simulink model "VentilatorActivity_Start"  (R2024b)
settings: Solver=VariableStepAuto  StartTime=0.0  StopTime=10.0  RelTol=1e-3
model workspace (MAT data in the model file):
  HeatCmd = Simulink.Bus
  HeatCmd.Alignment = -1
  HeatCmd.PreserveElementDimensions = 0
  HeatCmd.Elements_internal = Simulink.BusElement
  HeatCmd.Elements_internal.DimensionsMode = 'Fixed'
  HeatCmd.Elements_internal.SamplingMode = 'Sample based'
  HeatCmd.Elements_internal.SampleTime = -1
  HeatCmd.Elements_internal.Name = 'Element'
  HeatCmd.Elements_internal.DataType_internal = 'double'
  HeatCmd.Elements_internal.Complexity = 'real'
  HeatCmd.Elements_internal.Dimensions = 1
  HeatCmd.DataScope = 'Auto'
  HeaterCmd = Simulink.Bus
  HeaterCmd.Alignment = -1
  HeaterCmd.PreserveElementDimensions = 0
  HeaterCmd.DataScope = 'Auto'
  HumidSens = Simulink.Bus
  HumidSens.Alignment = -1
  HumidSens.PreserveElementDimensions = 0
  HumidSens.DataScope = 'Auto'
  init = Simulink.Bus
  init.Alignment = -1
  init.PreserveElementDimensions = 0
  init.DataScope = 'Auto'
settings Model: Creator=ppatel  LastModifiedBy=ppatel

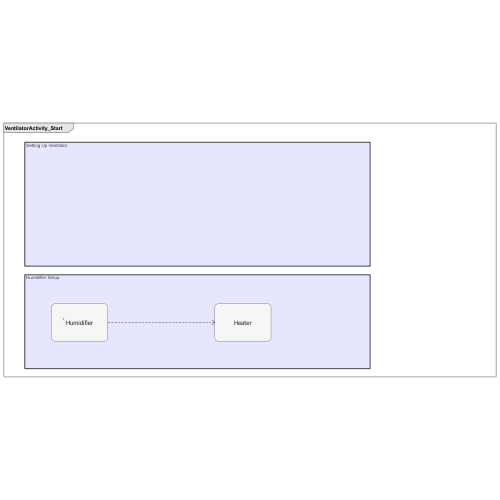
[thumbnail: Simulink's stored preview of the top-level diagram]
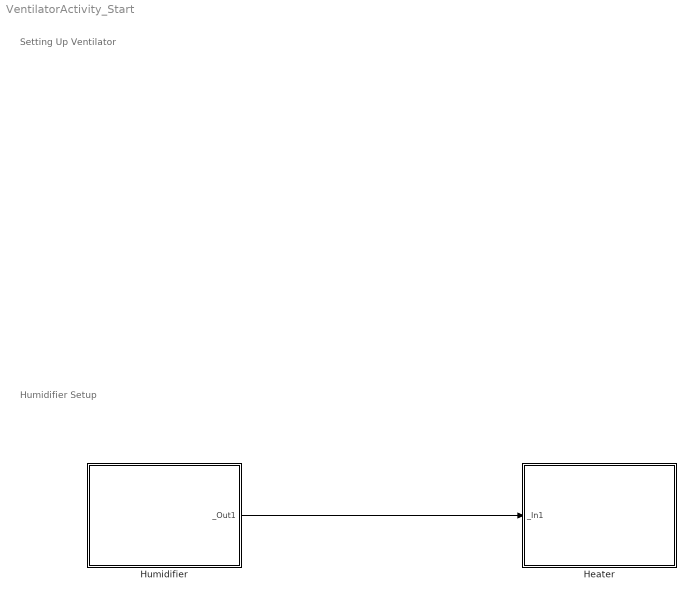
== system VentilatorActivity_Start ==
  note: Humidifier Setup
  note: Setting Up Ventilator
  Heater : Subsystem
      settings: CopyFcn=set_param(gcbh,'LinkStatus','none');  PortSchema="{\"entries\":[{\"content\":{\"sides\":[{\"content\":{\"connectorIds\":[\"In1\"]},\"type\":\"ConnectorPlacement.EquallySpacedRectSide\",\"uuid\":\"da638e69-4a2c-4548-ace4-820cc1f60a8d\"},{\"content\":{\"side\":\"RIGHT\"},\"type\":\"ConnectorPlacement.EquallySpacedRectSide\",\"uuid\":\"6a8a70e9-7f6e-4f36-a19f-a4054ca44662\"},{\"content\":{\"side\":\"TOP\"},\"type\":\"ConnectorPlacement.EquallySpacedRectSide\",\"uuid\":\"d1e931e2-f76e-4992-8014-0092805a8671\"}]},\"type\":\"ConnectorPlacement.EquallySpacedConnector\",\"uuid\":\"55c0ca13-68f0-475a-9ea9-fab942dd6d78\"}],\"packageUris\":[\"http://schema.mathworks.com/mf0/Connector/R2020b\"],\"version\":\"1.0\"}"
  Humidifier : Subsystem
      settings: CopyFcn=set_param(gcbh,'LinkStatus','none');  PortSchema="{\"entries\":[{\"content\":{\"sides\":[{\"content\":{},\"type\":\"ConnectorPlacement.EquallySpacedRectSide\",\"uuid\":\"da638e69-4a2c-4548-ace4-820cc1f60a8d\"},{\"content\":{\"connectorIds\":[\"Out1\"],\"side\":\"RIGHT\"},\"type\":\"ConnectorPlacement.EquallySpacedRectSide\",\"uuid\":\"6a8a70e9-7f6e-4f36-a19f-a4054ca44662\"},{\"content\":{\"side\":\"TOP\"},\"type\":\"ConnectorPlacement.EquallySpacedRectSide\",\"uuid\":\"d1e931e2-f76e-4992-8014-0092805a8671\"}]},\"type\":\"ConnectorPlacement.EquallySpacedConnector\",\"uuid\":\"55c0ca13-68f0-475a-9ea9-fab942dd6d78\"}],\"packageUris\":[\"http://schema.mathworks.com/mf0/Connector/R2020b\"],\"version\":\"1.0\"}"
  wires:
  Humidifier/1(_Out1) -> Heater/1(_In1)

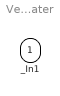
== system VentilatorActivity_Start/Heater ==
  _In1 : Inport

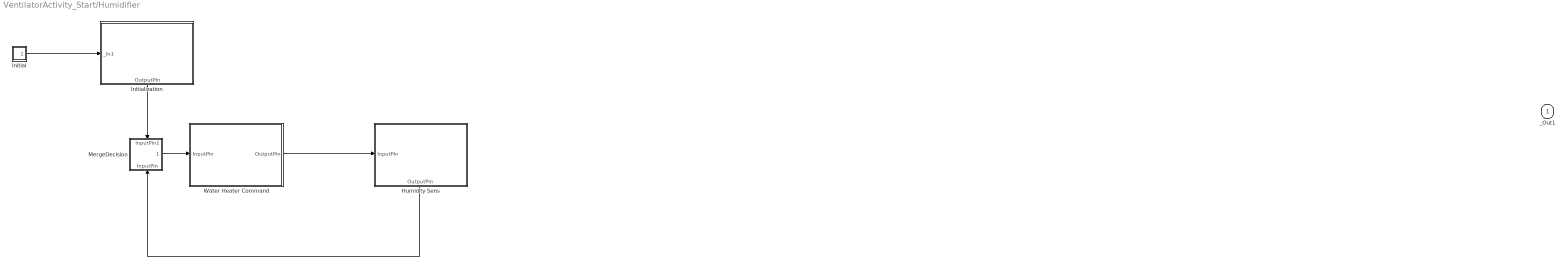
== system VentilatorActivity_Start/Humidifier ==
  Humidity Sens : Subsystem
      settings: CopyFcn=set_param(gcbh,'LinkStatus','none');  PortSchema="{\"entries\":[{\"content\":{\"sides\":[{\"content\":{\"connectorIds\":[\"In1\"]},\"type\":\"ConnectorPlacement.EquallySpacedRectSide\",\"uuid\":\"da638e69-4a2c-4548-ace4-820cc1f60a8d\"},{\"content\":{\"side\":\"RIGHT\"},\"type\":\"ConnectorPlacement.EquallySpacedRectSide\",\"uuid\":\"6a8a70e9-7f6e-4f36-a19f-a4054ca44662\"},{\"content\":{\"side\":\"TOP\"},\"type\":\"ConnectorPlacement.EquallySpacedRectSide\",\"uuid\":\"d1e931e2-f76e-4992-8014-0092805a8671\"},{\"content\":{\"connectorIds\":[\"Out1\"],\"side\":\"BOTTOM\"},\"type\":\"ConnectorPlacement.EquallySpacedRectSide\",\"uuid\":\"10984552-7b35-4f88-a27c-5daa08678015\"}]},\"type\":\"ConnectorPlacement.EquallySpacedConnector\",\"uuid\":\"55c0ca13-68f0-475a-9ea9-fab942dd6d78\"}],\"packageUris\":[\"http://schema.mathworks.com/mf0/Connector/R2020b\"],\"version\":\"1.0\"}"
  Initial : Subsystem
      settings: CopyFcn=set_param(gcbh,'LinkStatus','none');  PortSchema="{\"entries\":[{\"content\":{\"sides\":[{\"content\":{},\"type\":\"ConnectorPlacement.EquallySpacedRectSide\",\"uuid\":\"da638e69-4a2c-4548-ace4-820cc1f60a8d\"},{\"content\":{\"connectorIds\":[\"Out1\"],\"side\":\"RIGHT\"},\"type\":\"ConnectorPlacement.EquallySpacedRectSide\",\"uuid\":\"6a8a70e9-7f6e-4f36-a19f-a4054ca44662\"},{\"content\":{\"side\":\"TOP\"},\"type\":\"ConnectorPlacement.EquallySpacedRectSide\",\"uuid\":\"d1e931e2-f76e-4992-8014-0092805a8671\"}]},\"type\":\"ConnectorPlacement.EquallySpacedConnector\",\"uuid\":\"55c0ca13-68f0-475a-9ea9-fab942dd6d78\"}],\"packageUris\":[\"http://schema.mathworks.com/mf0/Connector/R2020b\"],\"version\":\"1.0\"}"
  Initialization : Subsystem
      settings: CopyFcn=set_param(gcbh,'LinkStatus','none');  PortSchema="{\"entries\":[{\"content\":{\"sides\":[{\"content\":{\"connectorIds\":[\"In1\"]},\"type\":\"ConnectorPlacement.EquallySpacedRectSide\",\"uuid\":\"da638e69-4a2c-4548-ace4-820cc1f60a8d\"},{\"content\":{\"side\":\"RIGHT\"},\"type\":\"ConnectorPlacement.EquallySpacedRectSide\",\"uuid\":\"6a8a70e9-7f6e-4f36-a19f-a4054ca44662\"},{\"content\":{\"side\":\"TOP\"},\"type\":\"ConnectorPlacement.EquallySpacedRectSide\",\"uuid\":\"d1e931e2-f76e-4992-8014-0092805a8671\"},{\"content\":{\"connectorIds\":[\"Out1\"],\"side\":\"BOTTOM\"},\"type\":\"ConnectorPlacement.EquallySpacedRectSide\",\"uuid\":\"856189ab-2e4f-4bf6-a759-2826ca9e7d61\"}]},\"type\":\"ConnectorPlacement.EquallySpacedConnector\",\"uuid\":\"55c0ca13-68f0-475a-9ea9-fab942dd6d78\"}],\"packageUris\":[\"http://schema.mathworks.com/mf0/Connector/R2020b\"],\"version\":\"1.0\"}"
  MergeDecision : Subsystem
      settings: CopyFcn=set_param(gcbh,'LinkStatus','none');  PortSchema="{\"entries\":[{\"content\":{\"sides\":[{\"content\":{},\"type\":\"ConnectorPlacement.EquallySpacedRectSide\",\"uuid\":\"da638e69-4a2c-4548-ace4-820cc1f60a8d\"},{\"content\":{\"connectorIds\":[\"Out1\"],\"side\":\"RIGHT\"},\"type\":\"ConnectorPlacement.EquallySpacedRectSide\",\"uuid\":\"6a8a70e9-7f6e-4f36-a19f-a4054ca44662\"},{\"content\":{\"connectorIds\":[\"In1\"],\"side\":\"TOP\"},\"type\":\"ConnectorPlacement.EquallySpacedRectSide\",\"uuid\":\"d1e931e2-f76e-4992-8014-0092805a8671\"},{\"content\":{\"connectorIds\":[\"In2\"],\"side\":\"BOTTOM\"},\"type\":\"ConnectorPlacement.EquallySpacedRectSide\",\"uuid\":\"1d127de0-f1c8-411a-9d19-34e7d29db091\"}]},\"type\":\"ConnectorPlacement.EquallySpacedConnector\",\"uuid\":\"55c0ca13-68f0-475a-9ea9-fab942dd6d78\"}],\"packageUris\":[\"http://schema.mathworks.com/mf0/Connector/R2020b\"],\"version\":\"1.0\"}"
  Water Heater Command : Subsystem
      settings: CopyFcn=set_param(gcbh,'LinkStatus','none');  PortSchema="{\"entries\":[{\"content\":{\"sides\":[{\"content\":{\"connectorIds\":[\"In1\"]},\"type\":\"ConnectorPlacement.EquallySpacedRectSide\",\"uuid\":\"da638e69-4a2c-4548-ace4-820cc1f60a8d\"},{\"content\":{\"connectorIds\":[\"Out1\"],\"side\":\"RIGHT\"},\"type\":\"ConnectorPlacement.EquallySpacedRectSide\",\"uuid\":\"6a8a70e9-7f6e-4f36-a19f-a4054ca44662\"},{\"content\":{\"side\":\"TOP\"},\"type\":\"ConnectorPlacement.EquallySpacedRectSide\",\"uuid\":\"d1e931e2-f76e-4992-8014-0092805a8671\"},{\"content\":{\"side\":\"BOTTOM\"},\"type\":\"ConnectorPlacement.EquallySpacedRectSide\",\"uuid\":\"c8c6cd51-bc28-4508-8599-fc70c851359e\"}]},\"type\":\"ConnectorPlacement.EquallySpacedConnector\",\"uuid\":\"55c0ca13-68f0-475a-9ea9-fab942dd6d78\"}],\"packageUris\":[\"http://schema.mathworks.com/mf0/Connector/R2020b\"],\"version\":\"1.0\"}"
  _Out1 : Outport
  wires:
  Water Heater Command/1(OutputPin) -> Humidity Sens/1(InputPin)
  Humidity Sens/1(OutputPin) -> MergeDecision/2(InputPin)
  MergeDecision/1(_Out1) -> Water Heater Command/1(InputPin)
  Initial/1(_Out1) -> Initialization/1(_In1)
  Initialization/1(OutputPin) -> MergeDecision/1(InputPin1)

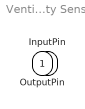
== system VentilatorActivity_Start/Humidifier/Humidity Sens ==
  InputPin : Inport
  OutputPin : Outport  OutDataTypeStr=double  PortDimensions=1

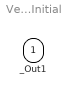
== system VentilatorActivity_Start/Humidifier/Initial ==
  _Out1 : Outport

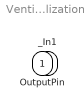
== system VentilatorActivity_Start/Humidifier/Initialization ==
  _In1 : Inport
  OutputPin : Outport  OutDataTypeStr=double  PortDimensions=1

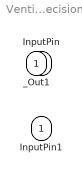
== system VentilatorActivity_Start/Humidifier/MergeDecision ==
  InputPin1 : Inport
  InputPin : Inport  Port=2
  _Out1 : Outport

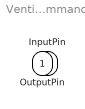
== system VentilatorActivity_Start/Humidifier/Water Heater Command ==
  InputPin : Inport
  OutputPin : Outport  OutDataTypeStr=double  PortDimensions=1
